simulink model "Modeling_three_phase_inverter"  (R2023b)
settings: Solver=ode1  StartTime=0.0  StopTime=1.5  FixedStep=2e-6  RelTol=1e-3
InitFcn:
  | warning('off','physmod:simscape:engine:core:advancer_errors:fallback_solve')
libraries: nesl_utility x22, fl_lib x20, ee_lib x14, sdl_lib x1, eePwmGenerator x1
(part 2 of 3)

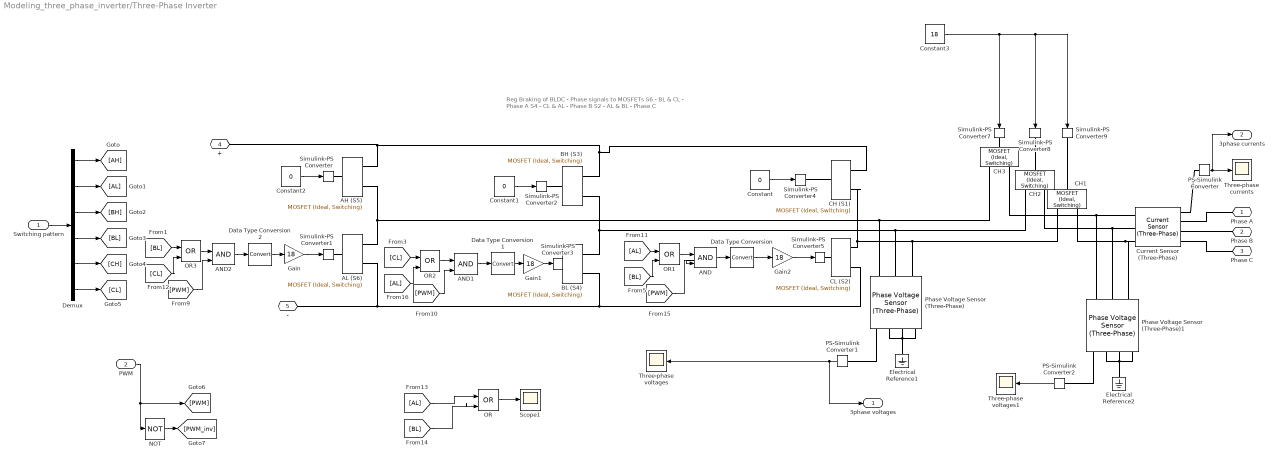
== system Modeling_three_phase_inverter/Three-Phase Inverter ==
  note: Reg Braking of BLDC - Phase signals to MOSFETs
      |
      | S6 - BL & CL - Phase A
      | S4 - CL & AL - Phase B
      | S2 - AL & BL - Phase C
  Switching pattern : Inport
  PWM : Inport  Port=2
  AH (S5) : ee_lib/Semiconductors & Converters/MOSFET (Ideal, Switching)  Tag={'toolbox/physmod/elec/library/m/ee_lib_parts';'Semiconductors_and_Converters/MOSFET__Ideal__Switching_/Infineon/IMZA120R007M1H.xml'}  port_option=ee.enum.controlport.ps  Rds=0.009 % Datasheet derived Ohm  Goff=2e-08 % Datasheet derived 1/Ohm  Vth=4.2 % Datasheet derived V  diode_param=ee.enum.converters.protectiondiode.nodynamics  diode_Vf=3.57 % Datasheet derived V  diode_Ron=0.008 % Datasheet derived Ohm  diode_Goff=1e-05 % Library default 1/Ohm  diode_C=50e-9 % Parameter not set F  diode_iRM=-235 % Parameter not set A  diode_iF=300 % Parameter not set A  diode_idot=-50 % Parameter not set A/us  diode_trr_param=ee.enum.converters.diodeReverseParam.trr_factor  diode_trr_factor=3 % Parameter not set  diode_trr=15 % Parameter not set us  diode_Qrr=1500 % Parameter not set s*uA  ids_specify=off  ids_priority=None  ids=0 A  ids_nominal_specify=off  ids_nominal_unit=A  ids_nominal_value=1  vds_specify=off  vds_priority=None  vds=0 V  vds_nominal_specify=off  vds_nominal_unit=V  vds_nominal_value=1  vgs_specify=off  vgs_priority=None  vgs=0 V  vgs_nominal_specify=off  vgs_nominal_unit=V  vgs_nominal_value=1  thermal_loss_option=ee.enum.converters.thermalLossOption.tabulated2d  Von_data=[0 0.38 0.76 1.15 1.55 1.95 2.35 2.74 3.13 3.51 3.9 4.34 4.8 5.26 5.71 6.17 6.63 7.09 7.61 8.17 8.73 9.28 9.97 10.67;0 0.81 1.62 2.43 3.22 4 4.79 5.61 6.42 7.23 8.06 8.9 9.74 10.59 11.48 12.38 13.29 14.19 15.08 15.96 16.87 17.85 18.82 19.79] % Datasheet derived V  Tj=[25 175] % Datasheet derived degC  Iout_data=[0 43.29 86.58 129.87 173.15 216.44 259.73 303.02 346.31 389.6 432.89 476.17 519.46 562.75 606.04 649.33 692.62 735.91 779.19 822.48 865.77 909.06 952.35 995.64] % Datasheet derived A  Eon_data=[353.65 402.32 450.99 499.66 548.33 597 645.67 694.34 743 791.67 840.34 889.01 937.68 986.35 1035.02 1083.69 1132.36 1181.03 1229.7 1278.37 1327.04 1375.71 1424.37 1473.04 1521.71 1570.38 1619.05 1667.72 1716.39 1765.06 1813.73 1862.4 1911.07 1959.91 2009.35 2058.79 2108.23 2157.67 2207.11 2256.56 2306 2355.44 2404.88 2454.32 2503.76 2553.21 2602.65 2652.09 2701.18 2748.37 2795.56 2842.74 2889.93 2937.12 2984.31 3031.5 3078.68 3125.87 3173.06 3220.25 3267.44 3314.62 3363.6 3413.28 3462.97 3512.66 3562.35 3612.03 3661.72 3711.41 3761.09 3810.78] % Datasheet derived uJ  Eoff_data=[203.9 211.68 219.47 227.25 235.04 242.82 250.61 258.39 266.18 273.96 281.74 289.53 297.31 305.1 312.88 320.67 328.45 336.24 344.02 351.8 359.59 367.37 375.16 382.94 390.73 398.51 406.3 414.08 421.87 429.65 437.43 445.22 453 460.79 468.57 476.36 484.14 491.93 499.38 506.77 514.15 521.54 528.93 536.32 543.71 551.1 558.49 565.88 573.27 580.66 588.04 595.43 602.82 610.21 617.42 624.45 631.48 638.51 645.54 652.57 659.59 666.62 673.65 680.68 687.71 694.74 701.76 708.79 715.82 722.85 729.88 736.91] % Datasheet derived uJ  Eon_data_3D=[zeros(2, 5, 3)] % Parameter not set J  Eoff_data_3D=[zeros(2, 5, 3)] % Parameter not set J  Tj_loss=175 % Datasheet derived degC  Iout_data_loss=[0 3.07 6.14 9.21 12.28 15.35 18.42 21.49 24.56 27.64 30.71 33.78 36.85 39.92 42.99 46.06 49.13 52.2 55.27 58.34 61.41 64.48 67.55 70.62 73.69 76.76 79.83 82.91 85.98 89.05 92.12 95.19 98.26 101.33 104.4 107.47 110.54 113.61 116.68 119.75 122.82 125.89 128.96 132.03 135.1 138.18 141.25 144.32 147.39 150.46 153.53 156.6 159.67 162.74 165.81 168.88 171.95 175.02 178.09 181.16 184.23 187.3 190.37 193.45 196.52 199.59 202.66 205.73 208.8 211.87 214.94 218.01] % Datasheet derived A  tabulateWithVds=false % Parameter not set  Vds_loss=[0, 150, 300] % Parameter not set V  Eon_scalar=22.86e-3 % Parameter not set J  Eoff_scalar=17.14e-3 % Parameter not set J  Voff=800 % Datasheet derived V  Iout_scalar=600 % Parameter not set A  useCurrentFromPreviousCycle=false  useVoltageFromPreviousCycle=false  diodeModelType=ee.enum.converters.diodeModelType.tabulated  diodeTableType=ee.enum.diode.tableType.IfMat  diode_IfMat=[0 0.5612 1.1331 1.9602 2.2 28.3686 98.5416 192.5511;0 0.9621 1.7462 2.2 10.5981 59.5348 141.4089 248.9] % Datasheet derived A  diode_VfMat=[.9, 1.15, 1.25, 1.5, 1.75, 2.17, 2.6, 2.85; .58, .68, .75, 1.1, 1.38, 1.77, 2.27, 2.7] % Parameter not set V  diode_TjVec=[25 175] % Datasheet derived degC  diode_VfVec=[0 0.86 1.71 2.57 3.43 4.29 5.14 6] % Datasheet derived V  diode_IfVec=[.1, .2, .5, 1, 2, 4, 7, 10] % Parameter not set A  diode_Vr=-600 % Parameter not set V  diode_Ls=150 % Parameter not set nH  diode_Erec=0.03 % Parameter not set J  diode_rec_loss_model=ee.enum.diode.reverseRecoveryModel.fixed  diode_ErecVal=0 % Parameter not set J  diode_scaleWithIandV=false  diode_ErecMat=zeros(2, 3) % Parameter not set J  diode_TjrecVec=[298.15, 398.15] % Parameter not set K  diode_IfrecVec=[.1, 1, 10] % Parameter not set A  diode_IrecVal=10 % Parameter not set A  diode_VrecVal=10 % Parameter not set V  diode_tFilter=1 / 1000 / 100 % Parameter not set s  thermal_network_parameterization=ee.enum.thermalNetworkTopology.external  Rth=[.03, .2] % Parameter not set K/W  Rth_Cauer=[.03, .1, .2] % Parameter not set K/W  Rth_Foster=[.03, .2] % Parameter not set K/W  thermal_mass_parameterization=ee.enum.thermalNetwork.timeconstant  thermal_mass=[3, 25] % Parameter not set J/K  thermal_mass_Cauer=[3, 10, 25] % Parameter not set J/K  thermal_mass_Foster=[33, 50] % Parameter not set J/K  thermal_time_constant=[.1, 5] % Parameter not set s  thermal_time_constant_Cauer=[.1, 1, 5] % Parameter not set s  thermal_time_constant_Foster=[1, 10] % Parameter not set s  thermal_mass_initial_temperatures=[25, 25] % Parameter not set degC  thermal_mass_initial_temperatures_Cauer=[25, 25, 25] % Parameter not set degC  junction_thermal_mass=4.04 % Datasheet derived J/K  Tvec_initial_Foster=[25, 25, 25, 25] % Parameter not set degC  no_thermal_network=0 % Parameter not set  junction_temperature_specify=off  junction_temperature_priority=None  junction_temperature=25 degC  junction_temperature_nominal_specify=off  junction_temperature_nominal_unit=degC  junction_temperature_nominal_value=1  Qj_specify=off  Qj_priority=None  Qj=0 W  Qj_nominal_specify=off  Qj_nominal_unit=W  Qj_nominal_value=1  accumulatedSwitchingLosses_specify=off  accumulatedSwitchingLosses_priority=None  accumulatedSwitchingLosses=0 J
      settings: AttributesFormatString=Infineon:IMZA120R007M1H
  AL (S6) : ee_lib/Semiconductors & Converters/MOSFET (Ideal, Switching)  Tag={'toolbox/physmod/elec/library/m/ee_lib_parts';'Semiconductors_and_Converters/MOSFET__Ideal__Switching_/Infineon/IMZA120R007M1H.xml'}  port_option=ee.enum.controlport.ps  Rds=0.009 % Datasheet derived Ohm  Goff=2e-08 % Datasheet derived 1/Ohm  Vth=4.2 % Datasheet derived V  diode_param=ee.enum.converters.protectiondiode.nodynamics  diode_Vf=3.57 % Datasheet derived V  diode_Ron=0.008 % Datasheet derived Ohm  diode_Goff=1e-05 % Library default 1/Ohm  diode_C=50e-9 % Parameter not set F  diode_iRM=-235 % Parameter not set A  diode_iF=300 % Parameter not set A  diode_idot=-50 % Parameter not set A/us  diode_trr_param=ee.enum.converters.diodeReverseParam.trr_factor  diode_trr_factor=3 % Parameter not set  diode_trr=15 % Parameter not set us  diode_Qrr=1500 % Parameter not set s*uA  ids_specify=off  ids_priority=None  ids=0 A  ids_nominal_specify=off  ids_nominal_unit=A  ids_nominal_value=1  vds_specify=off  vds_priority=None  vds=0 V  vds_nominal_specify=off  vds_nominal_unit=V  vds_nominal_value=1  vgs_specify=off  vgs_priority=None  vgs=0 V  vgs_nominal_specify=off  vgs_nominal_unit=V  vgs_nominal_value=1  thermal_loss_option=ee.enum.converters.thermalLossOption.tabulated2d  Von_data=[0 0.38 0.76 1.15 1.55 1.95 2.35 2.74 3.13 3.51 3.9 4.34 4.8 5.26 5.71 6.17 6.63 7.09 7.61 8.17 8.73 9.28 9.97 10.67;0 0.81 1.62 2.43 3.22 4 4.79 5.61 6.42 7.23 8.06 8.9 9.74 10.59 11.48 12.38 13.29 14.19 15.08 15.96 16.87 17.85 18.82 19.79] % Datasheet derived V  Tj=[25 175] % Datasheet derived degC  Iout_data=[0 43.29 86.58 129.87 173.15 216.44 259.73 303.02 346.31 389.6 432.89 476.17 519.46 562.75 606.04 649.33 692.62 735.91 779.19 822.48 865.77 909.06 952.35 995.64] % Datasheet derived A  Eon_data=[353.65 402.32 450.99 499.66 548.33 597 645.67 694.34 743 791.67 840.34 889.01 937.68 986.35 1035.02 1083.69 1132.36 1181.03 1229.7 1278.37 1327.04 1375.71 1424.37 1473.04 1521.71 1570.38 1619.05 1667.72 1716.39 1765.06 1813.73 1862.4 1911.07 1959.91 2009.35 2058.79 2108.23 2157.67 2207.11 2256.56 2306 2355.44 2404.88 2454.32 2503.76 2553.21 2602.65 2652.09 2701.18 2748.37 2795.56 2842.74 2889.93 2937.12 2984.31 3031.5 3078.68 3125.87 3173.06 3220.25 3267.44 3314.62 3363.6 3413.28 3462.97 3512.66 3562.35 3612.03 3661.72 3711.41 3761.09 3810.78] % Datasheet derived uJ  Eoff_data=[203.9 211.68 219.47 227.25 235.04 242.82 250.61 258.39 266.18 273.96 281.74 289.53 297.31 305.1 312.88 320.67 328.45 336.24 344.02 351.8 359.59 367.37 375.16 382.94 390.73 398.51 406.3 414.08 421.87 429.65 437.43 445.22 453 460.79 468.57 476.36 484.14 491.93 499.38 506.77 514.15 521.54 528.93 536.32 543.71 551.1 558.49 565.88 573.27 580.66 588.04 595.43 602.82 610.21 617.42 624.45 631.48 638.51 645.54 652.57 659.59 666.62 673.65 680.68 687.71 694.74 701.76 708.79 715.82 722.85 729.88 736.91] % Datasheet derived uJ  Eon_data_3D=[zeros(2, 5, 3)] % Parameter not set J  Eoff_data_3D=[zeros(2, 5, 3)] % Parameter not set J  Tj_loss=175 % Datasheet derived degC  Iout_data_loss=[0 3.07 6.14 9.21 12.28 15.35 18.42 21.49 24.56 27.64 30.71 33.78 36.85 39.92 42.99 46.06 49.13 52.2 55.27 58.34 61.41 64.48 67.55 70.62 73.69 76.76 79.83 82.91 85.98 89.05 92.12 95.19 98.26 101.33 104.4 107.47 110.54 113.61 116.68 119.75 122.82 125.89 128.96 132.03 135.1 138.18 141.25 144.32 147.39 150.46 153.53 156.6 159.67 162.74 165.81 168.88 171.95 175.02 178.09 181.16 184.23 187.3 190.37 193.45 196.52 199.59 202.66 205.73 208.8 211.87 214.94 218.01] % Datasheet derived A  tabulateWithVds=false % Parameter not set  Vds_loss=[0, 150, 300] % Parameter not set V  Eon_scalar=22.86e-3 % Parameter not set J  Eoff_scalar=17.14e-3 % Parameter not set J  Voff=800 % Datasheet derived V  Iout_scalar=600 % Parameter not set A  useCurrentFromPreviousCycle=false  useVoltageFromPreviousCycle=false  diodeModelType=ee.enum.converters.diodeModelType.tabulated  diodeTableType=ee.enum.diode.tableType.IfMat  diode_IfMat=[0 0.5612 1.1331 1.9602 2.2 28.3686 98.5416 192.5511;0 0.9621 1.7462 2.2 10.5981 59.5348 141.4089 248.9] % Datasheet derived A  diode_VfMat=[.9, 1.15, 1.25, 1.5, 1.75, 2.17, 2.6, 2.85; .58, .68, .75, 1.1, 1.38, 1.77, 2.27, 2.7] % Parameter not set V  diode_TjVec=[25 175] % Datasheet derived degC  diode_VfVec=[0 0.86 1.71 2.57 3.43 4.29 5.14 6] % Datasheet derived V  diode_IfVec=[.1, .2, .5, 1, 2, 4, 7, 10] % Parameter not set A  diode_Vr=-600 % Parameter not set V  diode_Ls=150 % Parameter not set nH  diode_Erec=0.03 % Parameter not set J  diode_rec_loss_model=ee.enum.diode.reverseRecoveryModel.fixed  diode_ErecVal=0 % Parameter not set J  diode_scaleWithIandV=false  diode_ErecMat=zeros(2, 3) % Parameter not set J  diode_TjrecVec=[298.15, 398.15] % Parameter not set K  diode_IfrecVec=[.1, 1, 10] % Parameter not set A  diode_IrecVal=10 % Parameter not set A  diode_VrecVal=10 % Parameter not set V  diode_tFilter=1 / 1000 / 100 % Parameter not set s  thermal_network_parameterization=ee.enum.thermalNetworkTopology.external  Rth=[.03, .2] % Parameter not set K/W  Rth_Cauer=[.03, .1, .2] % Parameter not set K/W  Rth_Foster=[.03, .2] % Parameter not set K/W  thermal_mass_parameterization=ee.enum.thermalNetwork.timeconstant  thermal_mass=[3, 25] % Parameter not set J/K  thermal_mass_Cauer=[3, 10, 25] % Parameter not set J/K  thermal_mass_Foster=[33, 50] % Parameter not set J/K  thermal_time_constant=[.1, 5] % Parameter not set s  thermal_time_constant_Cauer=[.1, 1, 5] % Parameter not set s  thermal_time_constant_Foster=[1, 10] % Parameter not set s  thermal_mass_initial_temperatures=[25, 25] % Parameter not set degC  thermal_mass_initial_temperatures_Cauer=[25, 25, 25] % Parameter not set degC  junction_thermal_mass=4.04 % Datasheet derived J/K  Tvec_initial_Foster=[25, 25, 25, 25] % Parameter not set degC  no_thermal_network=0 % Parameter not set  junction_temperature_specify=off  junction_temperature_priority=None  junction_temperature=25 degC  junction_temperature_nominal_specify=off  junction_temperature_nominal_unit=degC  junction_temperature_nominal_value=1  Qj_specify=off  Qj_priority=None  Qj=0 W  Qj_nominal_specify=off  Qj_nominal_unit=W  Qj_nominal_value=1  accumulatedSwitchingLosses_specify=off  accumulatedSwitchingLosses_priority=None  accumulatedSwitchingLosses=0 J
      settings: AttributesFormatString=Infineon:IMZA120R007M1H
  AND : Logic  IconShape=distinctive  AllPortsSameDT=off  OutDataTypeStr=boolean
  AND1 : Logic  IconShape=distinctive  AllPortsSameDT=off  OutDataTypeStr=boolean
  AND2 : Logic  IconShape=distinctive  AllPortsSameDT=off  OutDataTypeStr=boolean
  BH (S3) : ee_lib/Semiconductors & Converters/MOSFET (Ideal, Switching)  Tag={'toolbox/physmod/elec/library/m/ee_lib_parts';'Semiconductors_and_Converters/MOSFET__Ideal__Switching_/Infineon/IMZA120R007M1H.xml'}  port_option=ee.enum.controlport.ps  Rds=0.009 % Datasheet derived Ohm  Goff=2e-08 % Datasheet derived 1/Ohm  Vth=4.2 % Datasheet derived V  diode_param=ee.enum.converters.protectiondiode.nodynamics  diode_Vf=3.57 % Datasheet derived V  diode_Ron=0.008 % Datasheet derived Ohm  diode_Goff=1e-05 % Library default 1/Ohm  diode_C=50e-9 % Parameter not set F  diode_iRM=-235 % Parameter not set A  diode_iF=300 % Parameter not set A  diode_idot=-50 % Parameter not set A/us  diode_trr_param=ee.enum.converters.diodeReverseParam.trr_factor  diode_trr_factor=3 % Parameter not set  diode_trr=15 % Parameter not set us  diode_Qrr=1500 % Parameter not set s*uA  ids_specify=off  ids_priority=None  ids=0 A  ids_nominal_specify=off  ids_nominal_unit=A  ids_nominal_value=1  vds_specify=off  vds_priority=None  vds=0 V  vds_nominal_specify=off  vds_nominal_unit=V  vds_nominal_value=1  vgs_specify=off  vgs_priority=None  vgs=0 V  vgs_nominal_specify=off  vgs_nominal_unit=V  vgs_nominal_value=1  thermal_loss_option=ee.enum.converters.thermalLossOption.tabulated2d  Von_data=[0 0.38 0.76 1.15 1.55 1.95 2.35 2.74 3.13 3.51 3.9 4.34 4.8 5.26 5.71 6.17 6.63 7.09 7.61 8.17 8.73 9.28 9.97 10.67;0 0.81 1.62 2.43 3.22 4 4.79 5.61 6.42 7.23 8.06 8.9 9.74 10.59 11.48 12.38 13.29 14.19 15.08 15.96 16.87 17.85 18.82 19.79] % Datasheet derived V  Tj=[25 175] % Datasheet derived degC  Iout_data=[0 43.29 86.58 129.87 173.15 216.44 259.73 303.02 346.31 389.6 432.89 476.17 519.46 562.75 606.04 649.33 692.62 735.91 779.19 822.48 865.77 909.06 952.35 995.64] % Datasheet derived A  Eon_data=[353.65 402.32 450.99 499.66 548.33 597 645.67 694.34 743 791.67 840.34 889.01 937.68 986.35 1035.02 1083.69 1132.36 1181.03 1229.7 1278.37 1327.04 1375.71 1424.37 1473.04 1521.71 1570.38 1619.05 1667.72 1716.39 1765.06 1813.73 1862.4 1911.07 1959.91 2009.35 2058.79 2108.23 2157.67 2207.11 2256.56 2306 2355.44 2404.88 2454.32 2503.76 2553.21 2602.65 2652.09 2701.18 2748.37 2795.56 2842.74 2889.93 2937.12 2984.31 3031.5 3078.68 3125.87 3173.06 3220.25 3267.44 3314.62 3363.6 3413.28 3462.97 3512.66 3562.35 3612.03 3661.72 3711.41 3761.09 3810.78] % Datasheet derived uJ  Eoff_data=[203.9 211.68 219.47 227.25 235.04 242.82 250.61 258.39 266.18 273.96 281.74 289.53 297.31 305.1 312.88 320.67 328.45 336.24 344.02 351.8 359.59 367.37 375.16 382.94 390.73 398.51 406.3 414.08 421.87 429.65 437.43 445.22 453 460.79 468.57 476.36 484.14 491.93 499.38 506.77 514.15 521.54 528.93 536.32 543.71 551.1 558.49 565.88 573.27 580.66 588.04 595.43 602.82 610.21 617.42 624.45 631.48 638.51 645.54 652.57 659.59 666.62 673.65 680.68 687.71 694.74 701.76 708.79 715.82 722.85 729.88 736.91] % Datasheet derived uJ  Eon_data_3D=[zeros(2, 5, 3)] % Parameter not set J  Eoff_data_3D=[zeros(2, 5, 3)] % Parameter not set J  Tj_loss=175 % Datasheet derived degC  Iout_data_loss=[0 3.07 6.14 9.21 12.28 15.35 18.42 21.49 24.56 27.64 30.71 33.78 36.85 39.92 42.99 46.06 49.13 52.2 55.27 58.34 61.41 64.48 67.55 70.62 73.69 76.76 79.83 82.91 85.98 89.05 92.12 95.19 98.26 101.33 104.4 107.47 110.54 113.61 116.68 119.75 122.82 125.89 128.96 132.03 135.1 138.18 141.25 144.32 147.39 150.46 153.53 156.6 159.67 162.74 165.81 168.88 171.95 175.02 178.09 181.16 184.23 187.3 190.37 193.45 196.52 199.59 202.66 205.73 208.8 211.87 214.94 218.01] % Datasheet derived A  tabulateWithVds=false % Parameter not set  Vds_loss=[0, 150, 300] % Parameter not set V  Eon_scalar=22.86e-3 % Parameter not set J  Eoff_scalar=17.14e-3 % Parameter not set J  Voff=800 % Datasheet derived V  Iout_scalar=600 % Parameter not set A  useCurrentFromPreviousCycle=false  useVoltageFromPreviousCycle=false  diodeModelType=ee.enum.converters.diodeModelType.tabulated  diodeTableType=ee.enum.diode.tableType.IfMat  diode_IfMat=[0 0.5612 1.1331 1.9602 2.2 28.3686 98.5416 192.5511;0 0.9621 1.7462 2.2 10.5981 59.5348 141.4089 248.9] % Datasheet derived A  diode_VfMat=[.9, 1.15, 1.25, 1.5, 1.75, 2.17, 2.6, 2.85; .58, .68, .75, 1.1, 1.38, 1.77, 2.27, 2.7] % Parameter not set V  diode_TjVec=[25 175] % Datasheet derived degC  diode_VfVec=[0 0.86 1.71 2.57 3.43 4.29 5.14 6] % Datasheet derived V  diode_IfVec=[.1, .2, .5, 1, 2, 4, 7, 10] % Parameter not set A  diode_Vr=-600 % Parameter not set V  diode_Ls=150 % Parameter not set nH  diode_Erec=0.03 % Parameter not set J  diode_rec_loss_model=ee.enum.diode.reverseRecoveryModel.fixed  diode_ErecVal=0 % Parameter not set J  diode_scaleWithIandV=false  diode_ErecMat=zeros(2, 3) % Parameter not set J  diode_TjrecVec=[298.15, 398.15] % Parameter not set K  diode_IfrecVec=[.1, 1, 10] % Parameter not set A  diode_IrecVal=10 % Parameter not set A  diode_VrecVal=10 % Parameter not set V  diode_tFilter=1 / 1000 / 100 % Parameter not set s  thermal_network_parameterization=ee.enum.thermalNetworkTopology.external  Rth=[.03, .2] % Parameter not set K/W  Rth_Cauer=[.03, .1, .2] % Parameter not set K/W  Rth_Foster=[.03, .2] % Parameter not set K/W  thermal_mass_parameterization=ee.enum.thermalNetwork.timeconstant  thermal_mass=[3, 25] % Parameter not set J/K  thermal_mass_Cauer=[3, 10, 25] % Parameter not set J/K  thermal_mass_Foster=[33, 50] % Parameter not set J/K  thermal_time_constant=[.1, 5] % Parameter not set s  thermal_time_constant_Cauer=[.1, 1, 5] % Parameter not set s  thermal_time_constant_Foster=[1, 10] % Parameter not set s  thermal_mass_initial_temperatures=[25, 25] % Parameter not set degC  thermal_mass_initial_temperatures_Cauer=[25, 25, 25] % Parameter not set degC  junction_thermal_mass=4.04 % Datasheet derived J/K  Tvec_initial_Foster=[25, 25, 25, 25] % Parameter not set degC  no_thermal_network=0 % Parameter not set  junction_temperature_specify=off  junction_temperature_priority=None  junction_temperature=25 degC  junction_temperature_nominal_specify=off  junction_temperature_nominal_unit=degC  junction_temperature_nominal_value=1  Qj_specify=off  Qj_priority=None  Qj=0 W  Qj_nominal_specify=off  Qj_nominal_unit=W  Qj_nominal_value=1  accumulatedSwitchingLosses_specify=off  accumulatedSwitchingLosses_priority=None  accumulatedSwitchingLosses=0 J
      settings: AttributesFormatString=Infineon:IMZA120R007M1H
  BL (S4) : ee_lib/Semiconductors & Converters/MOSFET (Ideal, Switching)  Tag={'toolbox/physmod/elec/library/m/ee_lib_parts';'Semiconductors_and_Converters/MOSFET__Ideal__Switching_/Infineon/IMZA120R007M1H.xml'}  port_option=ee.enum.controlport.ps  Rds=0.009 % Datasheet derived Ohm  Goff=2e-08 % Datasheet derived 1/Ohm  Vth=4.2 % Datasheet derived V  diode_param=ee.enum.converters.protectiondiode.nodynamics  diode_Vf=3.57 % Datasheet derived V  diode_Ron=0.008 % Datasheet derived Ohm  diode_Goff=1e-05 % Library default 1/Ohm  diode_C=50e-9 % Parameter not set F  diode_iRM=-235 % Parameter not set A  diode_iF=300 % Parameter not set A  diode_idot=-50 % Parameter not set A/us  diode_trr_param=ee.enum.converters.diodeReverseParam.trr_factor  diode_trr_factor=3 % Parameter not set  diode_trr=15 % Parameter not set us  diode_Qrr=1500 % Parameter not set s*uA  ids_specify=off  ids_priority=None  ids=0 A  ids_nominal_specify=off  ids_nominal_unit=A  ids_nominal_value=1  vds_specify=off  vds_priority=None  vds=0 V  vds_nominal_specify=off  vds_nominal_unit=V  vds_nominal_value=1  vgs_specify=off  vgs_priority=None  vgs=0 V  vgs_nominal_specify=off  vgs_nominal_unit=V  vgs_nominal_value=1  thermal_loss_option=ee.enum.converters.thermalLossOption.tabulated2d  Von_data=[0 0.38 0.76 1.15 1.55 1.95 2.35 2.74 3.13 3.51 3.9 4.34 4.8 5.26 5.71 6.17 6.63 7.09 7.61 8.17 8.73 9.28 9.97 10.67;0 0.81 1.62 2.43 3.22 4 4.79 5.61 6.42 7.23 8.06 8.9 9.74 10.59 11.48 12.38 13.29 14.19 15.08 15.96 16.87 17.85 18.82 19.79] % Datasheet derived V  Tj=[25 175] % Datasheet derived degC  Iout_data=[0 43.29 86.58 129.87 173.15 216.44 259.73 303.02 346.31 389.6 432.89 476.17 519.46 562.75 606.04 649.33 692.62 735.91 779.19 822.48 865.77 909.06 952.35 995.64] % Datasheet derived A  Eon_data=[353.65 402.32 450.99 499.66 548.33 597 645.67 694.34 743 791.67 840.34 889.01 937.68 986.35 1035.02 1083.69 1132.36 1181.03 1229.7 1278.37 1327.04 1375.71 1424.37 1473.04 1521.71 1570.38 1619.05 1667.72 1716.39 1765.06 1813.73 1862.4 1911.07 1959.91 2009.35 2058.79 2108.23 2157.67 2207.11 2256.56 2306 2355.44 2404.88 2454.32 2503.76 2553.21 2602.65 2652.09 2701.18 2748.37 2795.56 2842.74 2889.93 2937.12 2984.31 3031.5 3078.68 3125.87 3173.06 3220.25 3267.44 3314.62 3363.6 3413.28 3462.97 3512.66 3562.35 3612.03 3661.72 3711.41 3761.09 3810.78] % Datasheet derived uJ  Eoff_data=[203.9 211.68 219.47 227.25 235.04 242.82 250.61 258.39 266.18 273.96 281.74 289.53 297.31 305.1 312.88 320.67 328.45 336.24 344.02 351.8 359.59 367.37 375.16 382.94 390.73 398.51 406.3 414.08 421.87 429.65 437.43 445.22 453 460.79 468.57 476.36 484.14 491.93 499.38 506.77 514.15 521.54 528.93 536.32 543.71 551.1 558.49 565.88 573.27 580.66 588.04 595.43 602.82 610.21 617.42 624.45 631.48 638.51 645.54 652.57 659.59 666.62 673.65 680.68 687.71 694.74 701.76 708.79 715.82 722.85 729.88 736.91] % Datasheet derived uJ  Eon_data_3D=[zeros(2, 5, 3)] % Parameter not set J  Eoff_data_3D=[zeros(2, 5, 3)] % Parameter not set J  Tj_loss=175 % Datasheet derived degC  Iout_data_loss=[0 3.07 6.14 9.21 12.28 15.35 18.42 21.49 24.56 27.64 30.71 33.78 36.85 39.92 42.99 46.06 49.13 52.2 55.27 58.34 61.41 64.48 67.55 70.62 73.69 76.76 79.83 82.91 85.98 89.05 92.12 95.19 98.26 101.33 104.4 107.47 110.54 113.61 116.68 119.75 122.82 125.89 128.96 132.03 135.1 138.18 141.25 144.32 147.39 150.46 153.53 156.6 159.67 162.74 165.81 168.88 171.95 175.02 178.09 181.16 184.23 187.3 190.37 193.45 196.52 199.59 202.66 205.73 208.8 211.87 214.94 218.01] % Datasheet derived A  tabulateWithVds=false % Parameter not set  Vds_loss=[0, 150, 300] % Parameter not set V  Eon_scalar=22.86e-3 % Parameter not set J  Eoff_scalar=17.14e-3 % Parameter not set J  Voff=800 % Datasheet derived V  Iout_scalar=600 % Parameter not set A  useCurrentFromPreviousCycle=false  useVoltageFromPreviousCycle=false  diodeModelType=ee.enum.converters.diodeModelType.tabulated  diodeTableType=ee.enum.diode.tableType.IfMat  diode_IfMat=[0 0.5612 1.1331 1.9602 2.2 28.3686 98.5416 192.5511;0 0.9621 1.7462 2.2 10.5981 59.5348 141.4089 248.9] % Datasheet derived A  diode_VfMat=[.9, 1.15, 1.25, 1.5, 1.75, 2.17, 2.6, 2.85; .58, .68, .75, 1.1, 1.38, 1.77, 2.27, 2.7] % Parameter not set V  diode_TjVec=[25 175] % Datasheet derived degC  diode_VfVec=[0 0.86 1.71 2.57 3.43 4.29 5.14 6] % Datasheet derived V  diode_IfVec=[.1, .2, .5, 1, 2, 4, 7, 10] % Parameter not set A  diode_Vr=-600 % Parameter not set V  diode_Ls=150 % Parameter not set nH  diode_Erec=0.03 % Parameter not set J  diode_rec_loss_model=ee.enum.diode.reverseRecoveryModel.fixed  diode_ErecVal=0 % Parameter not set J  diode_scaleWithIandV=false  diode_ErecMat=zeros(2, 3) % Parameter not set J  diode_TjrecVec=[298.15, 398.15] % Parameter not set K  diode_IfrecVec=[.1, 1, 10] % Parameter not set A  diode_IrecVal=10 % Parameter not set A  diode_VrecVal=10 % Parameter not set V  diode_tFilter=1 / 1000 / 100 % Parameter not set s  thermal_network_parameterization=ee.enum.thermalNetworkTopology.external  Rth=[.03, .2] % Parameter not set K/W  Rth_Cauer=[.03, .1, .2] % Parameter not set K/W  Rth_Foster=[.03, .2] % Parameter not set K/W  thermal_mass_parameterization=ee.enum.thermalNetwork.timeconstant  thermal_mass=[3, 25] % Parameter not set J/K  thermal_mass_Cauer=[3, 10, 25] % Parameter not set J/K  thermal_mass_Foster=[33, 50] % Parameter not set J/K  thermal_time_constant=[.1, 5] % Parameter not set s  thermal_time_constant_Cauer=[.1, 1, 5] % Parameter not set s  thermal_time_constant_Foster=[1, 10] % Parameter not set s  thermal_mass_initial_temperatures=[25, 25] % Parameter not set degC  thermal_mass_initial_temperatures_Cauer=[25, 25, 25] % Parameter not set degC  junction_thermal_mass=4.04 % Datasheet derived J/K  Tvec_initial_Foster=[25, 25, 25, 25] % Parameter not set degC  no_thermal_network=0 % Parameter not set  junction_temperature_specify=off  junction_temperature_priority=None  junction_temperature=25 degC  junction_temperature_nominal_specify=off  junction_temperature_nominal_unit=degC  junction_temperature_nominal_value=1  Qj_specify=off  Qj_priority=None  Qj=0 W  Qj_nominal_specify=off  Qj_nominal_unit=W  Qj_nominal_value=1  accumulatedSwitchingLosses_specify=off  accumulatedSwitchingLosses_priority=None  accumulatedSwitchingLosses=0 J
      settings: AttributesFormatString=Infineon:IMZA120R007M1H
  CH (S1) : ee_lib/Semiconductors & Converters/MOSFET (Ideal, Switching)  Tag={'toolbox/physmod/elec/library/m/ee_lib_parts';'Semiconductors_and_Converters/MOSFET__Ideal__Switching_/Infineon/IMZA120R007M1H.xml'}  port_option=ee.enum.controlport.ps  Rds=0.009 % Datasheet derived Ohm  Goff=2e-08 % Datasheet derived 1/Ohm  Vth=4.2 % Datasheet derived V  diode_param=ee.enum.converters.protectiondiode.nodynamics  diode_Vf=3.57 % Datasheet derived V  diode_Ron=0.008 % Datasheet derived Ohm  diode_Goff=1e-05 % Library default 1/Ohm  diode_C=50e-9 % Parameter not set F  diode_iRM=-235 % Parameter not set A  diode_iF=300 % Parameter not set A  diode_idot=-50 % Parameter not set A/us  diode_trr_param=ee.enum.converters.diodeReverseParam.trr_factor  diode_trr_factor=3 % Parameter not set  diode_trr=15 % Parameter not set us  diode_Qrr=1500 % Parameter not set s*uA  ids_specify=off  ids_priority=None  ids=0 A  ids_nominal_specify=off  ids_nominal_unit=A  ids_nominal_value=1  vds_specify=off  vds_priority=None  vds=0 V  vds_nominal_specify=off  vds_nominal_unit=V  vds_nominal_value=1  vgs_specify=off  vgs_priority=None  vgs=0 V  vgs_nominal_specify=off  vgs_nominal_unit=V  vgs_nominal_value=1  thermal_loss_option=ee.enum.converters.thermalLossOption.tabulated2d  Von_data=[0 0.38 0.76 1.15 1.55 1.95 2.35 2.74 3.13 3.51 3.9 4.34 4.8 5.26 5.71 6.17 6.63 7.09 7.61 8.17 8.73 9.28 9.97 10.67;0 0.81 1.62 2.43 3.22 4 4.79 5.61 6.42 7.23 8.06 8.9 9.74 10.59 11.48 12.38 13.29 14.19 15.08 15.96 16.87 17.85 18.82 19.79] % Datasheet derived V  Tj=[25 175] % Datasheet derived degC  Iout_data=[0 43.29 86.58 129.87 173.15 216.44 259.73 303.02 346.31 389.6 432.89 476.17 519.46 562.75 606.04 649.33 692.62 735.91 779.19 822.48 865.77 909.06 952.35 995.64] % Datasheet derived A  Eon_data=[353.65 402.32 450.99 499.66 548.33 597 645.67 694.34 743 791.67 840.34 889.01 937.68 986.35 1035.02 1083.69 1132.36 1181.03 1229.7 1278.37 1327.04 1375.71 1424.37 1473.04 1521.71 1570.38 1619.05 1667.72 1716.39 1765.06 1813.73 1862.4 1911.07 1959.91 2009.35 2058.79 2108.23 2157.67 2207.11 2256.56 2306 2355.44 2404.88 2454.32 2503.76 2553.21 2602.65 2652.09 2701.18 2748.37 2795.56 2842.74 2889.93 2937.12 2984.31 3031.5 3078.68 3125.87 3173.06 3220.25 3267.44 3314.62 3363.6 3413.28 3462.97 3512.66 3562.35 3612.03 3661.72 3711.41 3761.09 3810.78] % Datasheet derived uJ  Eoff_data=[203.9 211.68 219.47 227.25 235.04 242.82 250.61 258.39 266.18 273.96 281.74 289.53 297.31 305.1 312.88 320.67 328.45 336.24 344.02 351.8 359.59 367.37 375.16 382.94 390.73 398.51 406.3 414.08 421.87 429.65 437.43 445.22 453 460.79 468.57 476.36 484.14 491.93 499.38 506.77 514.15 521.54 528.93 536.32 543.71 551.1 558.49 565.88 573.27 580.66 588.04 595.43 602.82 610.21 617.42 624.45 631.48 638.51 645.54 652.57 659.59 666.62 673.65 680.68 687.71 694.74 701.76 708.79 715.82 722.85 729.88 736.91] % Datasheet derived uJ  Eon_data_3D=[zeros(2, 5, 3)] % Parameter not set J  Eoff_data_3D=[zeros(2, 5, 3)] % Parameter not set J  Tj_loss=175 % Datasheet derived degC  Iout_data_loss=[0 3.07 6.14 9.21 12.28 15.35 18.42 21.49 24.56 27.64 30.71 33.78 36.85 39.92 42.99 46.06 49.13 52.2 55.27 58.34 61.41 64.48 67.55 70.62 73.69 76.76 79.83 82.91 85.98 89.05 92.12 95.19 98.26 101.33 104.4 107.47 110.54 113.61 116.68 119.75 122.82 125.89 128.96 132.03 135.1 138.18 141.25 144.32 147.39 150.46 153.53 156.6 159.67 162.74 165.81 168.88 171.95 175.02 178.09 181.16 184.23 187.3 190.37 193.45 196.52 199.59 202.66 205.73 208.8 211.87 214.94 218.01] % Datasheet derived A  tabulateWithVds=false % Parameter not set  Vds_loss=[0, 150, 300] % Parameter not set V  Eon_scalar=22.86e-3 % Parameter not set J  Eoff_scalar=17.14e-3 % Parameter not set J  Voff=800 % Datasheet derived V  Iout_scalar=600 % Parameter not set A  useCurrentFromPreviousCycle=false  useVoltageFromPreviousCycle=false  diodeModelType=ee.enum.converters.diodeModelType.tabulated  diodeTableType=ee.enum.diode.tableType.IfMat  diode_IfMat=[0 0.5612 1.1331 1.9602 2.2 28.3686 98.5416 192.5511;0 0.9621 1.7462 2.2 10.5981 59.5348 141.4089 248.9] % Datasheet derived A  diode_VfMat=[.9, 1.15, 1.25, 1.5, 1.75, 2.17, 2.6, 2.85; .58, .68, .75, 1.1, 1.38, 1.77, 2.27, 2.7] % Parameter not set V  diode_TjVec=[25 175] % Datasheet derived degC  diode_VfVec=[0 0.86 1.71 2.57 3.43 4.29 5.14 6] % Datasheet derived V  diode_IfVec=[.1, .2, .5, 1, 2, 4, 7, 10] % Parameter not set A  diode_Vr=-600 % Parameter not set V  diode_Ls=150 % Parameter not set nH  diode_Erec=0.03 % Parameter not set J  diode_rec_loss_model=ee.enum.diode.reverseRecoveryModel.fixed  diode_ErecVal=0 % Parameter not set J  diode_scaleWithIandV=false  diode_ErecMat=zeros(2, 3) % Parameter not set J  diode_TjrecVec=[298.15, 398.15] % Parameter not set K  diode_IfrecVec=[.1, 1, 10] % Parameter not set A  diode_IrecVal=10 % Parameter not set A  diode_VrecVal=10 % Parameter not set V  diode_tFilter=1 / 1000 / 100 % Parameter not set s  thermal_network_parameterization=ee.enum.thermalNetworkTopology.external  Rth=[.03, .2] % Parameter not set K/W  Rth_Cauer=[.03, .1, .2] % Parameter not set K/W  Rth_Foster=[.03, .2] % Parameter not set K/W  thermal_mass_parameterization=ee.enum.thermalNetwork.timeconstant  thermal_mass=[3, 25] % Parameter not set J/K  thermal_mass_Cauer=[3, 10, 25] % Parameter not set J/K  thermal_mass_Foster=[33, 50] % Parameter not set J/K  thermal_time_constant=[.1, 5] % Parameter not set s  thermal_time_constant_Cauer=[.1, 1, 5] % Parameter not set s  thermal_time_constant_Foster=[1, 10] % Parameter not set s  thermal_mass_initial_temperatures=[25, 25] % Parameter not set degC  thermal_mass_initial_temperatures_Cauer=[25, 25, 25] % Parameter not set degC  junction_thermal_mass=4.04 % Datasheet derived J/K  Tvec_initial_Foster=[25, 25, 25, 25] % Parameter not set degC  no_thermal_network=0 % Parameter not set  junction_temperature_specify=off  junction_temperature_priority=None  junction_temperature=25 degC  junction_temperature_nominal_specify=off  junction_temperature_nominal_unit=degC  junction_temperature_nominal_value=1  Qj_specify=off  Qj_priority=None  Qj=0 W  Qj_nominal_specify=off  Qj_nominal_unit=W  Qj_nominal_value=1  accumulatedSwitchingLosses_specify=off  accumulatedSwitchingLosses_priority=None  accumulatedSwitchingLosses=0 J
      settings: AttributesFormatString=Infineon:IMZA120R007M1H
  CH1 : ee_lib/Semiconductors & Converters/MOSFET (Ideal, Switching)  Tag={'toolbox/physmod/elec/library/m/ee_lib_parts';'Semiconductors_and_Converters/MOSFET__Ideal__Switching_/Infineon/IMZA120R007M1H.xml'}  port_option=ee.enum.controlport.ps  Rds=0.009 % Datasheet derived Ohm  Goff=2e-08 % Datasheet derived 1/Ohm  Vth=4.2 % Datasheet derived V  diode_param=ee.enum.converters.protectiondiode.nodynamics  diode_Vf=3.57 % Datasheet derived V  diode_Ron=0.008 % Datasheet derived Ohm  diode_Goff=1e-05 % Library default 1/Ohm  diode_C=50e-9 % Parameter not set F  diode_iRM=-235 % Parameter not set A  diode_iF=300 % Parameter not set A  diode_idot=-50 % Parameter not set A/us  diode_trr_param=ee.enum.converters.diodeReverseParam.trr_factor  diode_trr_factor=3 % Parameter not set  diode_trr=15 % Parameter not set us  diode_Qrr=1500 % Parameter not set s*uA  ids_specify=off  ids_priority=None  ids=0 A  ids_nominal_specify=off  ids_nominal_unit=A  ids_nominal_value=1  vds_specify=off  vds_priority=None  vds=0 V  vds_nominal_specify=off  vds_nominal_unit=V  vds_nominal_value=1  vgs_specify=off  vgs_priority=None  vgs=0 V  vgs_nominal_specify=off  vgs_nominal_unit=V  vgs_nominal_value=1  thermal_loss_option=ee.enum.converters.thermalLossOption.tabulated2d  Von_data=[0 0.38 0.76 1.15 1.55 1.95 2.35 2.74 3.13 3.51 3.9 4.34 4.8 5.26 5.71 6.17 6.63 7.09 7.61 8.17 8.73 9.28 9.97 10.67;0 0.81 1.62 2.43 3.22 4 4.79 5.61 6.42 7.23 8.06 8.9 9.74 10.59 11.48 12.38 13.29 14.19 15.08 15.96 16.87 17.85 18.82 19.79] % Datasheet derived V  Tj=[25 175] % Datasheet derived degC  Iout_data=[0 43.29 86.58 129.87 173.15 216.44 259.73 303.02 346.31 389.6 432.89 476.17 519.46 562.75 606.04 649.33 692.62 735.91 779.19 822.48 865.77 909.06 952.35 995.64] % Datasheet derived A  Eon_data=[353.65 402.32 450.99 499.66 548.33 597 645.67 694.34 743 791.67 840.34 889.01 937.68 986.35 1035.02 1083.69 1132.36 1181.03 1229.7 1278.37 1327.04 1375.71 1424.37 1473.04 1521.71 1570.38 1619.05 1667.72 1716.39 1765.06 1813.73 1862.4 1911.07 1959.91 2009.35 2058.79 2108.23 2157.67 2207.11 2256.56 2306 2355.44 2404.88 2454.32 2503.76 2553.21 2602.65 2652.09 2701.18 2748.37 2795.56 2842.74 2889.93 2937.12 2984.31 3031.5 3078.68 3125.87 3173.06 3220.25 3267.44 3314.62 3363.6 3413.28 3462.97 3512.66 3562.35 3612.03 3661.72 3711.41 3761.09 3810.78] % Datasheet derived uJ  Eoff_data=[203.9 211.68 219.47 227.25 235.04 242.82 250.61 258.39 266.18 273.96 281.74 289.53 297.31 305.1 312.88 320.67 328.45 336.24 344.02 351.8 359.59 367.37 375.16 382.94 390.73 398.51 406.3 414.08 421.87 429.65 437.43 445.22 453 460.79 468.57 476.36 484.14 491.93 499.38 506.77 514.15 521.54 528.93 536.32 543.71 551.1 558.49 565.88 573.27 580.66 588.04 595.43 602.82 610.21 617.42 624.45 631.48 638.51 645.54 652.57 659.59 666.62 673.65 680.68 687.71 694.74 701.76 708.79 715.82 722.85 729.88 736.91] % Datasheet derived uJ  Eon_data_3D=[zeros(2, 5, 3)] % Parameter not set J  Eoff_data_3D=[zeros(2, 5, 3)] % Parameter not set J  Tj_loss=175 % Datasheet derived degC  Iout_data_loss=[0 3.07 6.14 9.21 12.28 15.35 18.42 21.49 24.56 27.64 30.71 33.78 36.85 39.92 42.99 46.06 49.13 52.2 55.27 58.34 61.41 64.48 67.55 70.62 73.69 76.76 79.83 82.91 85.98 89.05 92.12 95.19 98.26 101.33 104.4 107.47 110.54 113.61 116.68 119.75 122.82 125.89 128.96 132.03 135.1 138.18 141.25 144.32 147.39 150.46 153.53 156.6 159.67 162.74 165.81 168.88 171.95 175.02 178.09 181.16 184.23 187.3 190.37 193.45 196.52 199.59 202.66 205.73 208.8 211.87 214.94 218.01] % Datasheet derived A  tabulateWithVds=false % Parameter not set  Vds_loss=[0, 150, 300] % Parameter not set V  Eon_scalar=22.86e-3 % Parameter not set J  Eoff_scalar=17.14e-3 % Parameter not set J  Voff=800 % Datasheet derived V  Iout_scalar=600 % Parameter not set A  useCurrentFromPreviousCycle=false  useVoltageFromPreviousCycle=false  diodeModelType=ee.enum.converters.diodeModelType.tabulated  diodeTableType=ee.enum.diode.tableType.IfMat  diode_IfMat=[0 0.5612 1.1331 1.9602 2.2 28.3686 98.5416 192.5511;0 0.9621 1.7462 2.2 10.5981 59.5348 141.4089 248.9] % Datasheet derived A  diode_VfMat=[.9, 1.15, 1.25, 1.5, 1.75, 2.17, 2.6, 2.85; .58, .68, .75, 1.1, 1.38, 1.77, 2.27, 2.7] % Parameter not set V  diode_TjVec=[25 175] % Datasheet derived degC  diode_VfVec=[0 0.86 1.71 2.57 3.43 4.29 5.14 6] % Datasheet derived V  diode_IfVec=[.1, .2, .5, 1, 2, 4, 7, 10] % Parameter not set A  diode_Vr=-600 % Parameter not set V  diode_Ls=150 % Parameter not set nH  diode_Erec=0.03 % Parameter not set J  diode_rec_loss_model=ee.enum.diode.reverseRecoveryModel.fixed  diode_ErecVal=0 % Parameter not set J  diode_scaleWithIandV=false  diode_ErecMat=zeros(2, 3) % Parameter not set J  diode_TjrecVec=[298.15, 398.15] % Parameter not set K  diode_IfrecVec=[.1, 1, 10] % Parameter not set A  diode_IrecVal=10 % Parameter not set A  diode_VrecVal=10 % Parameter not set V  diode_tFilter=1 / 1000 / 100 % Parameter not set s  thermal_network_parameterization=ee.enum.thermalNetworkTopology.external  Rth=[.03, .2] % Parameter not set K/W  Rth_Cauer=[.03, .1, .2] % Parameter not set K/W  Rth_Foster=[.03, .2] % Parameter not set K/W  thermal_mass_parameterization=ee.enum.thermalNetwork.timeconstant  thermal_mass=[3, 25] % Parameter not set J/K  thermal_mass_Cauer=[3, 10, 25] % Parameter not set J/K  thermal_mass_Foster=[33, 50] % Parameter not set J/K  thermal_time_constant=[.1, 5] % Parameter not set s  thermal_time_constant_Cauer=[.1, 1, 5] % Parameter not set s  thermal_time_constant_Foster=[1, 10] % Parameter not set s  thermal_mass_initial_temperatures=[25, 25] % Parameter not set degC  thermal_mass_initial_temperatures_Cauer=[25, 25, 25] % Parameter not set degC  junction_thermal_mass=4.04 % Datasheet derived J/K  Tvec_initial_Foster=[25, 25, 25, 25] % Parameter not set degC  no_thermal_network=0 % Parameter not set  junction_temperature_specify=off  junction_temperature_priority=None  junction_temperature=25 degC  junction_temperature_nominal_specify=off  junction_temperature_nominal_unit=degC  junction_temperature_nominal_value=1  Qj_specify=off  Qj_priority=None  Qj=0 W  Qj_nominal_specify=off  Qj_nominal_unit=W  Qj_nominal_value=1  accumulatedSwitchingLosses_specify=off  accumulatedSwitchingLosses_priority=None  accumulatedSwitchingLosses=0 J
      settings: AttributesFormatString=Infineon:IMZA120R007M1H
  CH2 : ee_lib/Semiconductors & Converters/MOSFET (Ideal, Switching)  Tag={'toolbox/physmod/elec/library/m/ee_lib_parts';'Semiconductors_and_Converters/MOSFET__Ideal__Switching_/Infineon/IMZA120R007M1H.xml'}  port_option=ee.enum.controlport.ps  Rds=0.009 % Datasheet derived Ohm  Goff=2e-08 % Datasheet derived 1/Ohm  Vth=4.2 % Datasheet derived V  diode_param=ee.enum.converters.protectiondiode.nodynamics  diode_Vf=3.57 % Datasheet derived V  diode_Ron=0.008 % Datasheet derived Ohm  diode_Goff=1e-05 % Library default 1/Ohm  diode_C=50e-9 % Parameter not set F  diode_iRM=-235 % Parameter not set A  diode_iF=300 % Parameter not set A  diode_idot=-50 % Parameter not set A/us  diode_trr_param=ee.enum.converters.diodeReverseParam.trr_factor  diode_trr_factor=3 % Parameter not set  diode_trr=15 % Parameter not set us  diode_Qrr=1500 % Parameter not set s*uA  ids_specify=off  ids_priority=None  ids=0 A  ids_nominal_specify=off  ids_nominal_unit=A  ids_nominal_value=1  vds_specify=off  vds_priority=None  vds=0 V  vds_nominal_specify=off  vds_nominal_unit=V  vds_nominal_value=1  vgs_specify=off  vgs_priority=None  vgs=0 V  vgs_nominal_specify=off  vgs_nominal_unit=V  vgs_nominal_value=1  thermal_loss_option=ee.enum.converters.thermalLossOption.tabulated2d  Von_data=[0 0.38 0.76 1.15 1.55 1.95 2.35 2.74 3.13 3.51 3.9 4.34 4.8 5.26 5.71 6.17 6.63 7.09 7.61 8.17 8.73 9.28 9.97 10.67;0 0.81 1.62 2.43 3.22 4 4.79 5.61 6.42 7.23 8.06 8.9 9.74 10.59 11.48 12.38 13.29 14.19 15.08 15.96 16.87 17.85 18.82 19.79] % Datasheet derived V  Tj=[25 175] % Datasheet derived degC  Iout_data=[0 43.29 86.58 129.87 173.15 216.44 259.73 303.02 346.31 389.6 432.89 476.17 519.46 562.75 606.04 649.33 692.62 735.91 779.19 822.48 865.77 909.06 952.35 995.64] % Datasheet derived A  Eon_data=[353.65 402.32 450.99 499.66 548.33 597 645.67 694.34 743 791.67 840.34 889.01 937.68 986.35 1035.02 1083.69 1132.36 1181.03 1229.7 1278.37 1327.04 1375.71 1424.37 1473.04 1521.71 1570.38 1619.05 1667.72 1716.39 1765.06 1813.73 1862.4 1911.07 1959.91 2009.35 2058.79 2108.23 2157.67 2207.11 2256.56 2306 2355.44 2404.88 2454.32 2503.76 2553.21 2602.65 2652.09 2701.18 2748.37 2795.56 2842.74 2889.93 2937.12 2984.31 3031.5 3078.68 3125.87 3173.06 3220.25 3267.44 3314.62 3363.6 3413.28 3462.97 3512.66 3562.35 3612.03 3661.72 3711.41 3761.09 3810.78] % Datasheet derived uJ  Eoff_data=[203.9 211.68 219.47 227.25 235.04 242.82 250.61 258.39 266.18 273.96 281.74 289.53 297.31 305.1 312.88 320.67 328.45 336.24 344.02 351.8 359.59 367.37 375.16 382.94 390.73 398.51 406.3 414.08 421.87 429.65 437.43 445.22 453 460.79 468.57 476.36 484.14 491.93 499.38 506.77 514.15 521.54 528.93 536.32 543.71 551.1 558.49 565.88 573.27 580.66 588.04 595.43 602.82 610.21 617.42 624.45 631.48 638.51 645.54 652.57 659.59 666.62 673.65 680.68 687.71 694.74 701.76 708.79 715.82 722.85 729.88 736.91] % Datasheet derived uJ  Eon_data_3D=[zeros(2, 5, 3)] % Parameter not set J  Eoff_data_3D=[zeros(2, 5, 3)] % Parameter not set J  Tj_loss=175 % Datasheet derived degC  Iout_data_loss=[0 3.07 6.14 9.21 12.28 15.35 18.42 21.49 24.56 27.64 30.71 33.78 36.85 39.92 42.99 46.06 49.13 52.2 55.27 58.34 61.41 64.48 67.55 70.62 73.69 76.76 79.83 82.91 85.98 89.05 92.12 95.19 98.26 101.33 104.4 107.47 110.54 113.61 116.68 119.75 122.82 125.89 128.96 132.03 135.1 138.18 141.25 144.32 147.39 150.46 153.53 156.6 159.67 162.74 165.81 168.88 171.95 175.02 178.09 181.16 184.23 187.3 190.37 193.45 196.52 199.59 202.66 205.73 208.8 211.87 214.94 218.01] % Datasheet derived A  tabulateWithVds=false % Parameter not set  Vds_loss=[0, 150, 300] % Parameter not set V  Eon_scalar=22.86e-3 % Parameter not set J  Eoff_scalar=17.14e-3 % Parameter not set J  Voff=800 % Datasheet derived V  Iout_scalar=600 % Parameter not set A  useCurrentFromPreviousCycle=false  useVoltageFromPreviousCycle=false  diodeModelType=ee.enum.converters.diodeModelType.tabulated  diodeTableType=ee.enum.diode.tableType.IfMat  diode_IfMat=[0 0.5612 1.1331 1.9602 2.2 28.3686 98.5416 192.5511;0 0.9621 1.7462 2.2 10.5981 59.5348 141.4089 248.9] % Datasheet derived A  diode_VfMat=[.9, 1.15, 1.25, 1.5, 1.75, 2.17, 2.6, 2.85; .58, .68, .75, 1.1, 1.38, 1.77, 2.27, 2.7] % Parameter not set V  diode_TjVec=[25 175] % Datasheet derived degC  diode_VfVec=[0 0.86 1.71 2.57 3.43 4.29 5.14 6] % Datasheet derived V  diode_IfVec=[.1, .2, .5, 1, 2, 4, 7, 10] % Parameter not set A  diode_Vr=-600 % Parameter not set V  diode_Ls=150 % Parameter not set nH  diode_Erec=0.03 % Parameter not set J  diode_rec_loss_model=ee.enum.diode.reverseRecoveryModel.fixed  diode_ErecVal=0 % Parameter not set J  diode_scaleWithIandV=false  diode_ErecMat=zeros(2, 3) % Parameter not set J  diode_TjrecVec=[298.15, 398.15] % Parameter not set K  diode_IfrecVec=[.1, 1, 10] % Parameter not set A  diode_IrecVal=10 % Parameter not set A  diode_VrecVal=10 % Parameter not set V  diode_tFilter=1 / 1000 / 100 % Parameter not set s  thermal_network_parameterization=ee.enum.thermalNetworkTopology.external  Rth=[.03, .2] % Parameter not set K/W  Rth_Cauer=[.03, .1, .2] % Parameter not set K/W  Rth_Foster=[.03, .2] % Parameter not set K/W  thermal_mass_parameterization=ee.enum.thermalNetwork.timeconstant  thermal_mass=[3, 25] % Parameter not set J/K  thermal_mass_Cauer=[3, 10, 25] % Parameter not set J/K  thermal_mass_Foster=[33, 50] % Parameter not set J/K  thermal_time_constant=[.1, 5] % Parameter not set s  thermal_time_constant_Cauer=[.1, 1, 5] % Parameter not set s  thermal_time_constant_Foster=[1, 10] % Parameter not set s  thermal_mass_initial_temperatures=[25, 25] % Parameter not set degC  thermal_mass_initial_temperatures_Cauer=[25, 25, 25] % Parameter not set degC  junction_thermal_mass=4.04 % Datasheet derived J/K  Tvec_initial_Foster=[25, 25, 25, 25] % Parameter not set degC  no_thermal_network=0 % Parameter not set  junction_temperature_specify=off  junction_temperature_priority=None  junction_temperature=25 degC  junction_temperature_nominal_specify=off  junction_temperature_nominal_unit=degC  junction_temperature_nominal_value=1  Qj_specify=off  Qj_priority=None  Qj=0 W  Qj_nominal_specify=off  Qj_nominal_unit=W  Qj_nominal_value=1  accumulatedSwitchingLosses_specify=off  accumulatedSwitchingLosses_priority=None  accumulatedSwitchingLosses=0 J
      settings: AttributesFormatString=Infineon:IMZA120R007M1H
  CH3 : ee_lib/Semiconductors & Converters/MOSFET (Ideal, Switching)  Tag={'toolbox/physmod/elec/library/m/ee_lib_parts';'Semiconductors_and_Converters/MOSFET__Ideal__Switching_/Infineon/IMZA120R007M1H.xml'}  port_option=ee.enum.controlport.ps  Rds=0.009 % Datasheet derived Ohm  Goff=2e-08 % Datasheet derived 1/Ohm  Vth=4.2 % Datasheet derived V  diode_param=ee.enum.converters.protectiondiode.nodynamics  diode_Vf=3.57 % Datasheet derived V  diode_Ron=0.008 % Datasheet derived Ohm  diode_Goff=1e-05 % Library default 1/Ohm  diode_C=50e-9 % Parameter not set F  diode_iRM=-235 % Parameter not set A  diode_iF=300 % Parameter not set A  diode_idot=-50 % Parameter not set A/us  diode_trr_param=ee.enum.converters.diodeReverseParam.trr_factor  diode_trr_factor=3 % Parameter not set  diode_trr=15 % Parameter not set us  diode_Qrr=1500 % Parameter not set s*uA  ids_specify=off  ids_priority=None  ids=0 A  ids_nominal_specify=off  ids_nominal_unit=A  ids_nominal_value=1  vds_specify=off  vds_priority=None  vds=0 V  vds_nominal_specify=off  vds_nominal_unit=V  vds_nominal_value=1  vgs_specify=off  vgs_priority=None  vgs=0 V  vgs_nominal_specify=off  vgs_nominal_unit=V  vgs_nominal_value=1  thermal_loss_option=ee.enum.converters.thermalLossOption.tabulated2d  Von_data=[0 0.38 0.76 1.15 1.55 1.95 2.35 2.74 3.13 3.51 3.9 4.34 4.8 5.26 5.71 6.17 6.63 7.09 7.61 8.17 8.73 9.28 9.97 10.67;0 0.81 1.62 2.43 3.22 4 4.79 5.61 6.42 7.23 8.06 8.9 9.74 10.59 11.48 12.38 13.29 14.19 15.08 15.96 16.87 17.85 18.82 19.79] % Datasheet derived V  Tj=[25 175] % Datasheet derived degC  Iout_data=[0 43.29 86.58 129.87 173.15 216.44 259.73 303.02 346.31 389.6 432.89 476.17 519.46 562.75 606.04 649.33 692.62 735.91 779.19 822.48 865.77 909.06 952.35 995.64] % Datasheet derived A  Eon_data=[353.65 402.32 450.99 499.66 548.33 597 645.67 694.34 743 791.67 840.34 889.01 937.68 986.35 1035.02 1083.69 1132.36 1181.03 1229.7 1278.37 1327.04 1375.71 1424.37 1473.04 1521.71 1570.38 1619.05 1667.72 1716.39 1765.06 1813.73 1862.4 1911.07 1959.91 2009.35 2058.79 2108.23 2157.67 2207.11 2256.56 2306 2355.44 2404.88 2454.32 2503.76 2553.21 2602.65 2652.09 2701.18 2748.37 2795.56 2842.74 2889.93 2937.12 2984.31 3031.5 3078.68 3125.87 3173.06 3220.25 3267.44 3314.62 3363.6 3413.28 3462.97 3512.66 3562.35 3612.03 3661.72 3711.41 3761.09 3810.78] % Datasheet derived uJ  Eoff_data=[203.9 211.68 219.47 227.25 235.04 242.82 250.61 258.39 266.18 273.96 281.74 289.53 297.31 305.1 312.88 320.67 328.45 336.24 344.02 351.8 359.59 367.37 375.16 382.94 390.73 398.51 406.3 414.08 421.87 429.65 437.43 445.22 453 460.79 468.57 476.36 484.14 491.93 499.38 506.77 514.15 521.54 528.93 536.32 543.71 551.1 558.49 565.88 573.27 580.66 588.04 595.43 602.82 610.21 617.42 624.45 631.48 638.51 645.54 652.57 659.59 666.62 673.65 680.68 687.71 694.74 701.76 708.79 715.82 722.85 729.88 736.91] % Datasheet derived uJ  Eon_data_3D=[zeros(2, 5, 3)] % Parameter not set J  Eoff_data_3D=[zeros(2, 5, 3)] % Parameter not set J  Tj_loss=175 % Datasheet derived degC  Iout_data_loss=[0 3.07 6.14 9.21 12.28 15.35 18.42 21.49 24.56 27.64 30.71 33.78 36.85 39.92 42.99 46.06 49.13 52.2 55.27 58.34 61.41 64.48 67.55 70.62 73.69 76.76 79.83 82.91 85.98 89.05 92.12 95.19 98.26 101.33 104.4 107.47 110.54 113.61 116.68 119.75 122.82 125.89 128.96 132.03 135.1 138.18 141.25 144.32 147.39 150.46 153.53 156.6 159.67 162.74 165.81 168.88 171.95 175.02 178.09 181.16 184.23 187.3 190.37 193.45 196.52 199.59 202.66 205.73 208.8 211.87 214.94 218.01] % Datasheet derived A  tabulateWithVds=false % Parameter not set  Vds_loss=[0, 150, 300] % Parameter not set V  Eon_scalar=22.86e-3 % Parameter not set J  Eoff_scalar=17.14e-3 % Parameter not set J  Voff=800 % Datasheet derived V  Iout_scalar=600 % Parameter not set A  useCurrentFromPreviousCycle=false  useVoltageFromPreviousCycle=false  diodeModelType=ee.enum.converters.diodeModelType.tabulated  diodeTableType=ee.enum.diode.tableType.IfMat  diode_IfMat=[0 0.5612 1.1331 1.9602 2.2 28.3686 98.5416 192.5511;0 0.9621 1.7462 2.2 10.5981 59.5348 141.4089 248.9] % Datasheet derived A  diode_VfMat=[.9, 1.15, 1.25, 1.5, 1.75, 2.17, 2.6, 2.85; .58, .68, .75, 1.1, 1.38, 1.77, 2.27, 2.7] % Parameter not set V  diode_TjVec=[25 175] % Datasheet derived degC  diode_VfVec=[0 0.86 1.71 2.57 3.43 4.29 5.14 6] % Datasheet derived V  diode_IfVec=[.1, .2, .5, 1, 2, 4, 7, 10] % Parameter not set A  diode_Vr=-600 % Parameter not set V  diode_Ls=150 % Parameter not set nH  diode_Erec=0.03 % Parameter not set J  diode_rec_loss_model=ee.enum.diode.reverseRecoveryModel.fixed  diode_ErecVal=0 % Parameter not set J  diode_scaleWithIandV=false  diode_ErecMat=zeros(2, 3) % Parameter not set J  diode_TjrecVec=[298.15, 398.15] % Parameter not set K  diode_IfrecVec=[.1, 1, 10] % Parameter not set A  diode_IrecVal=10 % Parameter not set A  diode_VrecVal=10 % Parameter not set V  diode_tFilter=1 / 1000 / 100 % Parameter not set s  thermal_network_parameterization=ee.enum.thermalNetworkTopology.external  Rth=[.03, .2] % Parameter not set K/W  Rth_Cauer=[.03, .1, .2] % Parameter not set K/W  Rth_Foster=[.03, .2] % Parameter not set K/W  thermal_mass_parameterization=ee.enum.thermalNetwork.timeconstant  thermal_mass=[3, 25] % Parameter not set J/K  thermal_mass_Cauer=[3, 10, 25] % Parameter not set J/K  thermal_mass_Foster=[33, 50] % Parameter not set J/K  thermal_time_constant=[.1, 5] % Parameter not set s  thermal_time_constant_Cauer=[.1, 1, 5] % Parameter not set s  thermal_time_constant_Foster=[1, 10] % Parameter not set s  thermal_mass_initial_temperatures=[25, 25] % Parameter not set degC  thermal_mass_initial_temperatures_Cauer=[25, 25, 25] % Parameter not set degC  junction_thermal_mass=4.04 % Datasheet derived J/K  Tvec_initial_Foster=[25, 25, 25, 25] % Parameter not set degC  no_thermal_network=0 % Parameter not set  junction_temperature_specify=off  junction_temperature_priority=None  junction_temperature=25 degC  junction_temperature_nominal_specify=off  junction_temperature_nominal_unit=degC  junction_temperature_nominal_value=1  Qj_specify=off  Qj_priority=None  Qj=0 W  Qj_nominal_specify=off  Qj_nominal_unit=W  Qj_nominal_value=1  accumulatedSwitchingLosses_specify=off  accumulatedSwitchingLosses_priority=None  accumulatedSwitchingLosses=0 J
      settings: AttributesFormatString=Infineon:IMZA120R007M1H
  CL (S2) : ee_lib/Semiconductors & Converters/MOSFET (Ideal, Switching)  Tag={'toolbox/physmod/elec/library/m/ee_lib_parts';'Semiconductors_and_Converters/MOSFET__Ideal__Switching_/Infineon/IMZA120R007M1H.xml'}  port_option=ee.enum.controlport.ps  Rds=0.009 % Datasheet derived Ohm  Goff=2e-08 % Datasheet derived 1/Ohm  Vth=4.2 % Datasheet derived V  diode_param=ee.enum.converters.protectiondiode.nodynamics  diode_Vf=3.57 % Datasheet derived V  diode_Ron=0.008 % Datasheet derived Ohm  diode_Goff=1e-05 % Library default 1/Ohm  diode_C=50e-9 % Parameter not set F  diode_iRM=-235 % Parameter not set A  diode_iF=300 % Parameter not set A  diode_idot=-50 % Parameter not set A/us  diode_trr_param=ee.enum.converters.diodeReverseParam.trr_factor  diode_trr_factor=3 % Parameter not set  diode_trr=15 % Parameter not set us  diode_Qrr=1500 % Parameter not set s*uA  ids_specify=off  ids_priority=None  ids=0 A  ids_nominal_specify=off  ids_nominal_unit=A  ids_nominal_value=1  vds_specify=off  vds_priority=None  vds=0 V  vds_nominal_specify=off  vds_nominal_unit=V  vds_nominal_value=1  vgs_specify=off  vgs_priority=None  vgs=0 V  vgs_nominal_specify=off  vgs_nominal_unit=V  vgs_nominal_value=1  thermal_loss_option=ee.enum.converters.thermalLossOption.tabulated2d  Von_data=[0 0.38 0.76 1.15 1.55 1.95 2.35 2.74 3.13 3.51 3.9 4.34 4.8 5.26 5.71 6.17 6.63 7.09 7.61 8.17 8.73 9.28 9.97 10.67;0 0.81 1.62 2.43 3.22 4 4.79 5.61 6.42 7.23 8.06 8.9 9.74 10.59 11.48 12.38 13.29 14.19 15.08 15.96 16.87 17.85 18.82 19.79] % Datasheet derived V  Tj=[25 175] % Datasheet derived degC  Iout_data=[0 43.29 86.58 129.87 173.15 216.44 259.73 303.02 346.31 389.6 432.89 476.17 519.46 562.75 606.04 649.33 692.62 735.91 779.19 822.48 865.77 909.06 952.35 995.64] % Datasheet derived A  Eon_data=[353.65 402.32 450.99 499.66 548.33 597 645.67 694.34 743 791.67 840.34 889.01 937.68 986.35 1035.02 1083.69 1132.36 1181.03 1229.7 1278.37 1327.04 1375.71 1424.37 1473.04 1521.71 1570.38 1619.05 1667.72 1716.39 1765.06 1813.73 1862.4 1911.07 1959.91 2009.35 2058.79 2108.23 2157.67 2207.11 2256.56 2306 2355.44 2404.88 2454.32 2503.76 2553.21 2602.65 2652.09 2701.18 2748.37 2795.56 2842.74 2889.93 2937.12 2984.31 3031.5 3078.68 3125.87 3173.06 3220.25 3267.44 3314.62 3363.6 3413.28 3462.97 3512.66 3562.35 3612.03 3661.72 3711.41 3761.09 3810.78] % Datasheet derived uJ  Eoff_data=[203.9 211.68 219.47 227.25 235.04 242.82 250.61 258.39 266.18 273.96 281.74 289.53 297.31 305.1 312.88 320.67 328.45 336.24 344.02 351.8 359.59 367.37 375.16 382.94 390.73 398.51 406.3 414.08 421.87 429.65 437.43 445.22 453 460.79 468.57 476.36 484.14 491.93 499.38 506.77 514.15 521.54 528.93 536.32 543.71 551.1 558.49 565.88 573.27 580.66 588.04 595.43 602.82 610.21 617.42 624.45 631.48 638.51 645.54 652.57 659.59 666.62 673.65 680.68 687.71 694.74 701.76 708.79 715.82 722.85 729.88 736.91] % Datasheet derived uJ  Eon_data_3D=[zeros(2, 5, 3)] % Parameter not set J  Eoff_data_3D=[zeros(2, 5, 3)] % Parameter not set J  Tj_loss=175 % Datasheet derived degC  Iout_data_loss=[0 3.07 6.14 9.21 12.28 15.35 18.42 21.49 24.56 27.64 30.71 33.78 36.85 39.92 42.99 46.06 49.13 52.2 55.27 58.34 61.41 64.48 67.55 70.62 73.69 76.76 79.83 82.91 85.98 89.05 92.12 95.19 98.26 101.33 104.4 107.47 110.54 113.61 116.68 119.75 122.82 125.89 128.96 132.03 135.1 138.18 141.25 144.32 147.39 150.46 153.53 156.6 159.67 162.74 165.81 168.88 171.95 175.02 178.09 181.16 184.23 187.3 190.37 193.45 196.52 199.59 202.66 205.73 208.8 211.87 214.94 218.01] % Datasheet derived A  tabulateWithVds=false % Parameter not set  Vds_loss=[0, 150, 300] % Parameter not set V  Eon_scalar=22.86e-3 % Parameter not set J  Eoff_scalar=17.14e-3 % Parameter not set J  Voff=800 % Datasheet derived V  Iout_scalar=600 % Parameter not set A  useCurrentFromPreviousCycle=false  useVoltageFromPreviousCycle=false  diodeModelType=ee.enum.converters.diodeModelType.tabulated  diodeTableType=ee.enum.diode.tableType.IfMat  diode_IfMat=[0 0.5612 1.1331 1.9602 2.2 28.3686 98.5416 192.5511;0 0.9621 1.7462 2.2 10.5981 59.5348 141.4089 248.9] % Datasheet derived A  diode_VfMat=[.9, 1.15, 1.25, 1.5, 1.75, 2.17, 2.6, 2.85; .58, .68, .75, 1.1, 1.38, 1.77, 2.27, 2.7] % Parameter not set V  diode_TjVec=[25 175] % Datasheet derived degC  diode_VfVec=[0 0.86 1.71 2.57 3.43 4.29 5.14 6] % Datasheet derived V  diode_IfVec=[.1, .2, .5, 1, 2, 4, 7, 10] % Parameter not set A  diode_Vr=-600 % Parameter not set V  diode_Ls=150 % Parameter not set nH  diode_Erec=0.03 % Parameter not set J  diode_rec_loss_model=ee.enum.diode.reverseRecoveryModel.fixed  diode_ErecVal=0 % Parameter not set J  diode_scaleWithIandV=false  diode_ErecMat=zeros(2, 3) % Parameter not set J  diode_TjrecVec=[298.15, 398.15] % Parameter not set K  diode_IfrecVec=[.1, 1, 10] % Parameter not set A  diode_IrecVal=10 % Parameter not set A  diode_VrecVal=10 % Parameter not set V  diode_tFilter=1 / 1000 / 100 % Parameter not set s  thermal_network_parameterization=ee.enum.thermalNetworkTopology.external  Rth=[.03, .2] % Parameter not set K/W  Rth_Cauer=[.03, .1, .2] % Parameter not set K/W  Rth_Foster=[.03, .2] % Parameter not set K/W  thermal_mass_parameterization=ee.enum.thermalNetwork.timeconstant  thermal_mass=[3, 25] % Parameter not set J/K  thermal_mass_Cauer=[3, 10, 25] % Parameter not set J/K  thermal_mass_Foster=[33, 50] % Parameter not set J/K  thermal_time_constant=[.1, 5] % Parameter not set s  thermal_time_constant_Cauer=[.1, 1, 5] % Parameter not set s  thermal_time_constant_Foster=[1, 10] % Parameter not set s  thermal_mass_initial_temperatures=[25, 25] % Parameter not set degC  thermal_mass_initial_temperatures_Cauer=[25, 25, 25] % Parameter not set degC  junction_thermal_mass=4.04 % Datasheet derived J/K  Tvec_initial_Foster=[25, 25, 25, 25] % Parameter not set degC  no_thermal_network=0 % Parameter not set  junction_temperature_specify=off  junction_temperature_priority=None  junction_temperature=25 degC  junction_temperature_nominal_specify=off  junction_temperature_nominal_unit=degC  junction_temperature_nominal_value=1  Qj_specify=off  Qj_priority=None  Qj=0 W  Qj_nominal_specify=off  Qj_nominal_unit=W  Qj_nominal_value=1  accumulatedSwitchingLosses_specify=off  accumulatedSwitchingLosses_priority=None  accumulatedSwitchingLosses=0 J
      settings: AttributesFormatString=Infineon:IMZA120R007M1H
  Constant : Constant  Value=0
  Constant1 : Constant  Value=0
  Constant2 : Constant  Value=0
  Constant3 : Constant  Value=18
  Current Sensor (Three-Phase) : ee_lib/Sensors & Transducers/Current Sensor (Three-Phase)
      settings: InternalSimscapePortConfiguration="{\"Bottom\":[],\"Left\":[{\"id\":\"a1\",\"label\":\"a1\",\"type\":\"foundation.electrical.electrical\"},{\"id\":\"b1\",\"label\":\"b1\",\"type\":\"foundation.electrical.electrical\"},{\"id\":\"c1\",\"label\":\"c1\",\"type\":\"foundation.electrical.electrical\"}],\"Right\":[{\"id\":\"I_output\",\"label\":\"I\",\"type\":\"output\"},{\"id\":\"a2\",\"label\":\"a2\",\"type\":\"foundation.electrical.electrical\"},{\"id\":\"b2\",\"label\":\"b2\",\"type\":\"foundation.electrical.electrical\"},{\"id\":\"c2\",\"label\":\"c2\",\"type\":\"foundation.electrical.electrical\"}],\"Top\":[]}"
  Data Type Conversion : DataTypeConversion  SaturateOnIntegerOverflow=off  RndMeth=Floor
  Data Type Conversion1 : DataTypeConversion  SaturateOnIntegerOverflow=off  RndMeth=Floor
  Data Type Conversion2 : DataTypeConversion  SaturateOnIntegerOverflow=off  RndMeth=Floor
  Demux : Demux  Outputs=6
  Electrical Reference1 : fl_lib/Electrical/Electrical Elements/Electrical Reference
  Electrical Reference2 : fl_lib/Electrical/Electrical Elements/Electrical Reference
  Gain : Gain  Gain=18
  Gain1 : Gain  Gain=18
  Gain2 : Gain  Gain=18
  NOT : Logic  Operator=NOT  IconShape=distinctive  AllPortsSameDT=off  OutDataTypeStr=boolean
  OR{,1..3} (4 alike) : Logic  Operator=OR  IconShape=distinctive  AllPortsSameDT=off  OutDataTypeStr=boolean
  PS-Simulink Converter : nesl_utility/PS-Simulink Converter  PhysicalDomain=network_engine_domain  SubClassName=ps_output  LeftPortType=input  RightPortType=output  PseudoPeriodic=off  Frequencies=[]  VectorFormat=1-D array  Unit=1  AffineConversion=off
  PS-Simulink Converter1 : nesl_utility/PS-Simulink Converter  PhysicalDomain=network_engine_domain  SubClassName=ps_output  LeftPortType=input  RightPortType=output  PseudoPeriodic=off  Frequencies=[]  VectorFormat=1-D array  Unit=1  AffineConversion=off
  PS-Simulink Converter2 : nesl_utility/PS-Simulink Converter  PhysicalDomain=network_engine_domain  SubClassName=ps_output  LeftPortType=input  RightPortType=output  PseudoPeriodic=off  Frequencies=[]  VectorFormat=1-D array  Unit=1  AffineConversion=off
  Phase Voltage Sensor (Three-Phase) : ee_lib/Sensors & Transducers/Phase Voltage Sensor (Three-Phase)
      settings: InternalSimscapePortConfiguration="{\"Bottom\":[],\"Left\":[{\"id\":\"a1\",\"label\":\"a1\",\"type\":\"foundation.electrical.electrical\"},{\"id\":\"b1\",\"label\":\"b1\",\"type\":\"foundation.electrical.electrical\"},{\"id\":\"c1\",\"label\":\"c1\",\"type\":\"foundation.electrical.electrical\"}],\"Right\":[{\"id\":\"V_output\",\"label\":\"V\",\"type\":\"output\"},{\"id\":\"a2\",\"label\":\"a2\",\"type\":\"foundation.electrical.electrical\"},{\"id\":\"b2\",\"label\":\"b2\",\"type\":\"foundation.electrical.electrical\"},{\"id\":\"c2\",\"label\":\"c2\",\"type\":\"foundation.electrical.electrical\"}],\"Top\":[]}"
  Phase Voltage Sensor (Three-Phase)1 : ee_lib/Sensors & Transducers/Phase Voltage Sensor (Three-Phase)
      settings: InternalSimscapePortConfiguration="{\"Bottom\":[],\"Left\":[{\"id\":\"a1\",\"label\":\"a1\",\"type\":\"foundation.electrical.electrical\"},{\"id\":\"b1\",\"label\":\"b1\",\"type\":\"foundation.electrical.electrical\"},{\"id\":\"c1\",\"label\":\"c1\",\"type\":\"foundation.electrical.electrical\"}],\"Right\":[{\"id\":\"V_output\",\"label\":\"V\",\"type\":\"output\"},{\"id\":\"a2\",\"label\":\"a2\",\"type\":\"foundation.electrical.electrical\"},{\"id\":\"b2\",\"label\":\"b2\",\"type\":\"foundation.electrical.electrical\"},{\"id\":\"c2\",\"label\":\"c2\",\"type\":\"foundation.electrical.electrical\"}],\"Top\":[]}"
  Scope1 : Scope
  Simulink-PS Converter{,1..5,7..9} (9 alike) : nesl_utility/Simulink-PS Converter  PhysicalDomain=network_engine_domain  SubClassName=ps_input  LeftPortType=input  RightPortType=output  PseudoPeriodic=off  Frequencies=[]  NoiseDistribution=none  NoiseParameters=[]  Unit=1  AffineConversion=off  FilteringAndDerivatives=provide  SimscapeFilterOrder=1  InputFilterTimeConstant=0.001  UdotUserProvided=0
  Three-phase currents : Scope
  Three-phase voltages : Scope
  Three-phase voltages1 : Scope
  Phase A : PMIOPort  Side=Right
  Phase B : PMIOPort  Port=2  Side=Right
  Phase C : PMIOPort  Port=3  Side=Right
  + : PMIOPort  Port=4  Side=Left
  - : PMIOPort  Port=5  Side=Left
  3phase voltages : Outport
  3phase currents : Outport  Port=2
  wires:
  Switching pattern/1 -> Demux/1
  Demux/1 -> [AH]
  Demux/5 -> [CH]
  Demux/4 -> [BL]
  Demux/3 -> [BH]
  Demux/2 -> [AL]
  Demux/6 -> [CL]
  PS-Simulink Converter1/1 -> 3phase voltages/1, Three-phase voltages/1
  PS-Simulink Converter/1 -> 3phase currents/1, Three-phase currents/1
  [BL] -> OR1/2
  [AL] -> OR1/1
  PS-Simulink Converter2/1 -> Three-phase voltages1/1
  NOT/1 -> [PWM_inv]
  [AL] -> OR/1
  [BL] -> OR/2
  OR/1 -> Scope1/1
  OR1/1 -> AND/1
  [PWM] -> AND/2
  OR2/1 -> AND1/1
  [PWM] -> AND1/2
  [CL] -> OR2/1
  [AL] -> OR2/2
  OR3/1 -> AND2/1
  [PWM] -> AND2/2
  [BL] -> OR3/1
  [CL] -> OR3/2
  Data Type Conversion/1 -> Gain2/1
  AND/1 -> Data Type Conversion/1
  Data Type Conversion1/1 -> Gain1/1
  AND1/1 -> Data Type Conversion1/1
  AND2/1 -> Data Type Conversion2/1
  Data Type Conversion2/1 -> Gain/1
  Constant/1 -> Simulink-PS Converter4/1
  Constant1/1 -> Simulink-PS Converter2/1
  Constant2/1 -> Simulink-PS Converter/1
  Constant3/1 -> Simulink-PS Converter7/1, Simulink-PS Converter8/1, Simulink-PS Converter9/1
  PWM/1 -> [PWM], NOT/1
  Gain/1 -> Simulink-PS Converter1/1
  Gain1/1 -> Simulink-PS Converter3/1
  Gain2/1 -> Simulink-PS Converter5/1
  connections:
  CH (S1)/RConn1 -- BH (S3)/RConn1 -- +/RConn1 -- AH (S5)/RConn1
  Phase Voltage Sensor (Three-Phase)/RConn3 -- Phase Voltage Sensor (Three-Phase)/RConn4 -- Phase Voltage Sensor (Three-Phase)/RConn2 -- Electrical Reference1/LConn1
  Current Sensor (Three-Phase)/RConn3 -- Phase B/RConn1
  Simulink-PS Converter3/RConn1 -- BL (S4)/LConn1
  Current Sensor (Three-Phase)/RConn4 -- Phase C/RConn1
  AH (S5)/RConn2 -- CH3/RConn2 -- Phase Voltage Sensor (Three-Phase)/LConn1 -- AL (S6)/RConn1
  AL (S6)/RConn2 -- CL (S2)/RConn2 -- BL (S4)/RConn2 -- -/RConn1
  Simulink-PS Converter5/RConn1 -- CL (S2)/LConn1
  CH (S1)/RConn2 -- CH1/RConn2 -- Phase Voltage Sensor (Three-Phase)/LConn3 -- CL (S2)/RConn1
  Simulink-PS Converter4/RConn1 -- CH (S1)/LConn1
  PS-Simulink Converter1/LConn1 -- Phase Voltage Sensor (Three-Phase)/RConn1
  Simulink-PS Converter/RConn1 -- AH (S5)/LConn1
  Current Sensor (Three-Phase)/RConn2 -- Phase A/RConn1
  Simulink-PS Converter1/RConn1 -- AL (S6)/LConn1
  Current Sensor (Three-Phase)/RConn1 -- PS-Simulink Converter/LConn1
  Simulink-PS Converter2/RConn1 -- BH (S3)/LConn1
  CH3/RConn1 -- Phase Voltage Sensor (Three-Phase)1/LConn1 -- Current Sensor (Three-Phase)/LConn1
  CH2/RConn1 -- Phase Voltage Sensor (Three-Phase)1/LConn2 -- Current Sensor (Three-Phase)/LConn2
  Current Sensor (Three-Phase)/LConn3 -- Phase Voltage Sensor (Three-Phase)1/LConn3 -- CH1/RConn1
  Electrical Reference2/LConn1 -- Phase Voltage Sensor (Three-Phase)1/RConn3 -- Phase Voltage Sensor (Three-Phase)1/RConn4 -- Phase Voltage Sensor (Three-Phase)1/RConn2
  PS-Simulink Converter2/LConn1 -- Phase Voltage Sensor (Three-Phase)1/RConn1
  BH (S3)/RConn2 -- BL (S4)/RConn1 -- CH2/RConn2 -- Phase Voltage Sensor (Three-Phase)/LConn2
  Simulink-PS Converter7/RConn1 -- CH3/LConn1
  Simulink-PS Converter9/RConn1 -- CH1/LConn1
  Simulink-PS Converter8/RConn1 -- CH2/LConn1
